simulink model "inAndOut_25b"  (R2025b)
settings: Solver=VariableStepAuto  AbsTol=1e-3
undefined symbols (not defined in the file or in its folder): ee_sli_rtmsupport, gcbh
libraries: nesl_utility x8
settings Model: Creator=yifany  LastModifiedBy=yifany
settings SolverCC: AutoScaleAbsTol=off  AlgebraicLoopSolver=TrustRegion  MaxZcPerStep=1.0
settings DebuggingCC: UnconnectedInputMsg=warning  UnconnectedOutputMsg=warning  UnconnectedLineMsg=warning  SymbolicDimsDataTypeCodeGenerationDiagnostic=none
settings ModelReferenceCC: EnableRefExpFcnMdlSchedulingChecks=on
settings SFSimCC: CustomCodeUndefinedFunction=UseInterfaceOnly
settings RTWCC: GPUComputeCapability=3.5  DLArmComputeVersion=19.05
settings SimscapeCC: SimscapeLogType=all  SimscapeLogSimulationStatistics=on  SimscapeLogDataHistory=10000.0

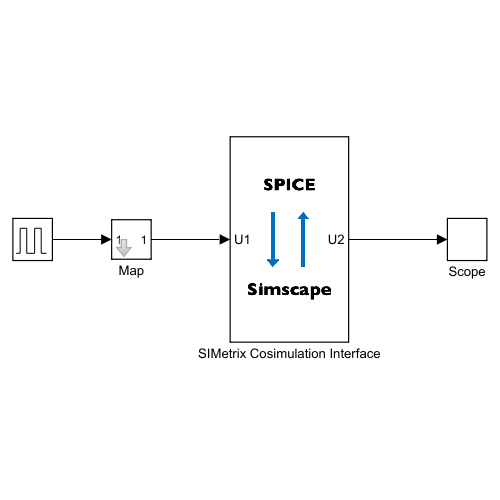
[thumbnail: Simulink's stored preview of the top-level diagram]
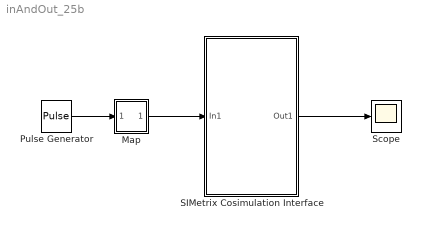
== system inAndOut_25b ==
  Map : Subsystem  mask{mapInput0=-8, mapInput1=25}
      mask prompts: mapInput0 "Map input 0 to output"; mapInput1 "Map input 1 to output"
      mask DialogControl DescTextVar Prompt: Linear map the input to the output
      mask DialogControl map Prompt: Map
  Pulse Generator : DiscretePulseGenerator  PulseType=Time based  Period=0.1  PulseWidth=40
  SIMetrix Cosimulation Interface : Subsystem  LoadFcn=ee_sli_rtmsupport( 'loadfcn', gcbh );  InitFcn=|  mask(SIMetrix Co-Simulation Interface){netlistFilePath=C:\Users\yifany\OneDrive - MathWorks\Desktop\Co-simulation\25b\inAndOut.net, flagGenerateInterface=1, numInputs=6, numOutputs=0, numVoltage=3, numCurrent=0, sampleTime=1e-3, updateIcon=1, DLLPath=C:\Program Files\SIMetrix910\bin64\Slif.dll}
      | % Checks Windows and sets the DLL path
      | ee.spice.internal.setDLLPathForWindows(gcb)
      mask prompts: netlistFilePath "physmod:ee:cosimulation:NetlistFilePath_MP"; numInputs "Number of simulink input signals"; numOutputs "Number of simulink output signals"; numVoltage "Number of voltage source electrical ports"; numCurrent "Number of current source electrical ports"; sampleTime "physmod:ee:cosimulation:SampleTime_MP"; updateIcon "Update Icon"; DLLPath "DLL path"
      mask help: physmod:ee:cosimulation:SimetrixCosimulationInterfacesBlock_MD
      mask init:
      | % Create the mask obj
      | maskObj = ee.spice.mask.cosimSIMetrix(gcb);
      | % Build IO
      | maskObj.buildIO;
      settings: DeleteFcn=ee_sli_rtmsupport( 'deletefcn', gcbh );  ModelCloseFcn=ee_sli_rtmsupport( 'modelclosefcn', gcbh );  PostSaveFcn=ee_sli_rtmsupport( 'postsavefcn', gcbh );  PreCopyFcn=ee_sli_rtmsupport( 'precopyfcn', gcbh );  OpenFcn=ee_sli_rtmsupport( 'openfcn', gcbh );  CloseFcn=ee_sli_rtmsupport( 'closefcn', gcbh );  PreDeleteFcn=ee_sli_rtmsupport( 'predeletefcn', gcbh );
      settings: CopyFcn=|
      | set_param(gcb,'LinkStatus','none')
      | ee_sli_rtmsupport( 'copyfcn', gcbh );
      mask Help: web([docroot '/sps/ref/simetrixcosimulationinterface.html'])
      mask DialogControl netlistFilePath Prompt: Netlist file path
      mask DialogControl BrowseBtn Prompt: physmod:ee:cosimulation:Browse_MP
      mask DialogControl BrowseBtn Callback:
      | % Create the mask obj
      | maskObj = ee.spice.mask.cosimSIMetrix(gcb);
      | % Browse netlist path
      | maskObj.browseNetlistPath;
      mask DialogControl buildIO Prompt: physmod:ee:cosimulation:BuildIO_MP
      mask DialogControl buildIO Callback:
      | blockObj = get_param(gcb,'Object');
      | dlg = DAStudio.ToolRoot.getOpenDialogs(blockObj.getDialogSource);
      | if ~isempty(dlg)
      |     dlg.apply;
      | end
      mask DialogControl numIO Prompt: I/O number
      mask DialogControl sampleTime Prompt: Sample time
      mask Display:
      | image('cosimSIMetrix.svg');
      | 
      | % Get parameters
      | updateIcon = str2double(get_param(gcb, 'updateIcon'));
      | netlistFilePath = get_param(gcb, 'netlistFilePath');
      | 
      | % Get interface port information from the netlist
      | if updateIcon
      |     netlistObj = ee.spice.internal.interfacePortInfo(netlistFilePath);
      |      % Get port information from the netlsit
      |      netlistObj = netlistObj.getPortsFromNetlist;
      | else
      |     netlistObj = ee.spice.internal.interfacePortInfo([]);
      | end
      | 
      | % Interface port handle
      | portHandles = get_param(gcb, 'PortHandles');
      | 
      | % Add input label
      | % Number of interface inport
      | numInport = length(portHandles.Inport);
      | for ii = 1:netlistObj.NumberOfInputs
      |     portName = upper(netlistObj.InputPortName(ii));
      |     if ii <= numInport
      |         port_label('input', ii, portName);
      |     end
      | end
      | 
      | % Add output label
      | % Number of interface outport
      | numOutport = length(portHandles.Outport);
      | for ii = 1:netlistObj.NumberOfOutputs
      |     portName = upper(netlistObj.OutputPortName(ii));
      |     if ii <= numOutport
      |         port_label('output', ii, portName);
      |     end
      | end
      | 
      | % Number of electrical connection port
      | numConnection = length(portHandles.RConn);
      | 
      | % Add voltage source electrical node
      | portIndex = 1;
      | for ii = 1:netlistObj.NumberOfVoltageSource
      |     portName = upper(netlistObj.VoltagePortName(ii));
      |     if netlistObj.VoltageIsDifferentialVector
      |         % Differential-end
      |         if portIndex + 1 <= numConnection
      |             port_label('rconn', portIndex, portName + "V +");
      |             port_label('rconn', portIndex + 1, portName + "V -");
      |             portIndex = portIndex + 2;
      |         end
      |     else
      |         % Single-end
      |         if portIndex <= numConnection
      |             port_label('rconn', portIndex, portName + "V");
      |             portIndex = portIndex + 1;
      |         end
      |     end
      | end
      | 
      | % Add current source electrical node
      | for ii = 1:netlistObj.NumberOfCurrentSource
      |     portName = upper(netlistObj.CurrentPortName(ii));
      |     if netlistObj.CurrentIsDifferentialVector
      |         % Differential-end
      |         if portIndex + 1 <= numConnection
      |             port_label('rconn', portIndex, portName + "I +");
      |             port_label('rconn', portIndex + 1, portName + "I -");
      |             portIndex = portIndex + 2;
      |         end
      |     else
      |         % Single-end
      |         if portIndex <= numConnection
      |             port_label('rconn', portIndex, portName + "I");
      |             portIndex = portIndex + 1;
      |         end
      |     end
      | end
  Scope : Scope
      settings: ActiveDisplayYMinimum=-61.816763160075034  ActiveDisplayYMaximum=562.41300067487691
  wires:
  SIMetrix Cosimulation Interface/1(Out1) -> Scope/1
  Pulse Generator/1 -> Map/1(In1)
  Map/1(Out1) -> SIMetrix Cosimulation Interface/1(In1)

== system inAndOut_25b/Map ==
  In1 : Inport
  Bias : Bias  Bias=mapInput0  SaturateOnIntegerOverflow=off
  Gain : Gain  Gain=mapInput1-mapInput0
  Out1 : Outport
  wires:
  Bias/1 -> Out1/1
  Gain/1 -> Bias/1
  In1/1 -> Gain/1

== system inAndOut_25b/SIMetrix Cosimulation Interface ==
  In1 : Inport
  Differential-Ended Network Coupler : Subsystem  Commented=on  Variant=on  mask{isNetworkCoupler=on, isVoltage=1, sampleTime=sampleTime, numNodes=1, i0=0, v0=0}
      mask prompts: isNetworkCoupler "Is network coupler"; isVoltage "Source type (1=voltage,0=current)"; sampleTime "Sample time (s)"; numNodes "Electrical node array size"; i0 "Initial current (A)"; v0 "Initial voltage (V)"
      settings: PortSchema="{\"entries\":[{\"content\":{\"sides\":[{\"content\":{\"connectorIds\":[\"In1\",\"Out1\"]},\"type\":\"ConnectorPlacement.EquallySpacedRectSide\",\"uuid\":\"c5b0d662-d741-4fab-bdd1-a9a465f659d9\"},{\"content\":{\"connectorIds\":[\"RConn1\",\"RConn2\"],\"side\":\"RIGHT\"},\"type\":\"ConnectorPlacement.EquallySpacedRectSide\",\"uuid\":\"848af5b9-7b7a-436a-bf47-17010bd721d3\"},{\"content\":{\"side\":\"TOP\"},\"type\":\"ConnectorPlacement.EquallySpacedRectSide\",\"uuid\":\"f4ff35f8-3dfd-4ab3-8ede-deadd7697822\"}]},\"type\":\"ConnectorPlacement.EquallySpacedConnector\",\"uuid\":\"b98b5658-49ee-4ac6-ad55-f0a4b59e49ca\"}],\"packageUris\":[\"http://schema.mathworks.com/mf0/Connector/R2020b\"],\"version\":\"1.0\"}"
      mask DialogControl DescGroupVar Prompt: Differential-Ended Network Coupler
      mask DialogControl DescTextVar Prompt: Connect Simscape differential electrical node pair(s) to SPICE via a controlled source.
      mask DialogControl Main Prompt: Main
      mask DialogControl InitialConditions Prompt: Initial Conditions
  S-function Interface to SIMetrix : S-Function  FunctionName=callSIMetrixInterface  Parameters=sampleTime, numInputs , elementsInput, numOutputs, elementsOutput, netlistPath, DLLPath  SFunctionDeploymentMode=off  EnableBusSupport=off  mask{sampleTime=sampleTime, numInputs=1, elementsInput=1, numOutputs=1, elementsOutput=1, netlistPath=C:\Users\yifany\OneDrive - MathWorks\Desktop\Co-simulation\25b\inAndOut.net, DLLPath=C:\Program Files\SIMetrix910\bin64\Slif.dll}
      mask prompts: sampleTime "Sample time (s)"; numInputs "Number of input ports"; elementsInput "Number of elements in each input"; numOutputs "Number of output ports"; elementsOutput "Number of elements in each output"; netlistPath "Netlist file path"; DLLPath "DLL path"
      mask init:
      | label = char(['Sample Time = ' num2str(sampleTime) 's']);
      mask Display: disp(label);
  Single-Ended Network Coupler : Subsystem  Commented=on  Variant=on  mask{isNetworkCoupler=on, isVoltage=1, sampleTime=sampleTime, numNodes=1, i0=0, v0=0}
      mask prompts: isNetworkCoupler "Is network coupler"; isVoltage "Source type (1=voltage,0=current)"; sampleTime "Sample time (s)"; numNodes "Electrical node array size"; i0 "Initial current (A)"; v0 "Initial voltage (V)"
      settings: PortSchema="{\"entries\":[{\"content\":{\"sides\":[{\"content\":{\"connectorIds\":[\"In1\",\"Out1\"]},\"type\":\"ConnectorPlacement.EquallySpacedRectSide\",\"uuid\":\"c5b0d662-d741-4fab-bdd1-a9a465f659d9\"},{\"content\":{\"connectorIds\":[\"RConn1\"],\"side\":\"RIGHT\"},\"type\":\"ConnectorPlacement.EquallySpacedRectSide\",\"uuid\":\"848af5b9-7b7a-436a-bf47-17010bd721d3\"},{\"content\":{\"side\":\"TOP\"},\"type\":\"ConnectorPlacement.EquallySpacedRectSide\",\"uuid\":\"f4ff35f8-3dfd-4ab3-8ede-deadd7697822\"}]},\"type\":\"ConnectorPlacement.EquallySpacedConnector\",\"uuid\":\"b98b5658-49ee-4ac6-ad55-f0a4b59e49ca\"}],\"packageUris\":[\"http://schema.mathworks.com/mf0/Connector/R2020b\"],\"version\":\"1.0\"}"
      mask DialogControl DescGroupVar Prompt: Network Single-End Coupler
      mask DialogControl DescTextVar Prompt: Connect Simscape single-ended electrical node(s) to SPICE via a controlled source.
      mask DialogControl Main Prompt: Main
      mask DialogControl InitialConditions Prompt: Initial Conditions
  Out1 : Outport
  wires:
  In1/1 -> S-function Interface to SIMetrix/1
  S-function Interface to SIMetrix/1 -> Out1/1

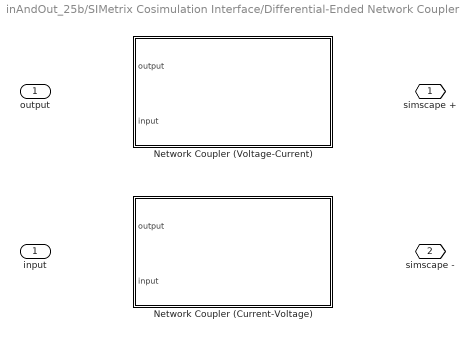
== system inAndOut_25b/SIMetrix Cosimulation Interface/Differential-Ended Network Coupler ==
  output : Inport
  Network Coupler (Current-Voltage) : Subsystem  VariantControl=isVoltage == 1  mask(SPICE-Simscape Interface (SPICE voltage source, Simscape current source)){h1=sampleTime, numNodes=numNodes, i0=i0, v0=v0}
      mask prompts: h1 "Sample time (s)"; numNodes "Electrical node array size"; i0 "Initial current (A)"; v0 "Initial voltage (V)"
      settings: PortSchema="{\"entries\":[{\"content\":{\"sides\":[{\"content\":{\"connectorIds\":[\"In1\",\"Out1\"]},\"type\":\"ConnectorPlacement.EquallySpacedRectSide\",\"uuid\":\"610a1ed6-b291-4a0b-a90d-70b8561de4e1\"},{\"content\":{\"connectorIds\":[\"RConn1\",\"RConn2\"],\"side\":\"RIGHT\"},\"type\":\"ConnectorPlacement.EquallySpacedRectSide\",\"uuid\":\"4485c82c-8fe2-4682-bcbc-6cb09abb17ba\"},{\"content\":{\"side\":\"TOP\"},\"type\":\"ConnectorPlacement.EquallySpacedRectSide\",\"uuid\":\"95b8fac6-4c79-4ea5-805e-3e8ec8ddf6c6\"}]},\"type\":\"ConnectorPlacement.EquallySpacedConnector\",\"uuid\":\"68c5dfd4-aae4-4799-81d8-d79fe9f653e9\"}],\"packageUris\":[\"http://schema.mathworks.com/mf0/Connector/R2020b\"],\"version\":\"1.0\"}"
      mask DialogControl Main Prompt: Main
      mask DialogControl InitialConditions Prompt: Initial Conditions
  Network Coupler (Voltage-Current) : Subsystem  VariantControl=isVoltage ~= 1  mask(SPICE-Simscape Interface (SPICE voltage source, Simscape current source)){h1=sampleTime, numNodes=numNodes, i0=i0, v0=v0}
      mask prompts: h1 "Sample time (s)"; numNodes "Electrical node array size"; i0 "Initial current (A)"; v0 "Initial voltage (V)"
      settings: PortSchema="{\"entries\":[{\"content\":{\"sides\":[{\"content\":{\"connectorIds\":[\"In1\",\"Out1\"]},\"type\":\"ConnectorPlacement.EquallySpacedRectSide\",\"uuid\":\"610a1ed6-b291-4a0b-a90d-70b8561de4e1\"},{\"content\":{\"connectorIds\":[\"RConn1\",\"RConn2\"],\"side\":\"RIGHT\"},\"type\":\"ConnectorPlacement.EquallySpacedRectSide\",\"uuid\":\"4485c82c-8fe2-4682-bcbc-6cb09abb17ba\"},{\"content\":{\"side\":\"TOP\"},\"type\":\"ConnectorPlacement.EquallySpacedRectSide\",\"uuid\":\"95b8fac6-4c79-4ea5-805e-3e8ec8ddf6c6\"}]},\"type\":\"ConnectorPlacement.EquallySpacedConnector\",\"uuid\":\"68c5dfd4-aae4-4799-81d8-d79fe9f653e9\"}],\"packageUris\":[\"http://schema.mathworks.com/mf0/Connector/R2020b\"],\"version\":\"1.0\"}"
      mask DialogControl Main Prompt: Main
      mask DialogControl InitialConditions Prompt: Initial Conditions
  simscape + : PMIOPort  Side=Right
  simscape - : PMIOPort  Port=2  Side=Right
  input : Outport

== system inAndOut_25b/SIMetrix Cosimulation Interface/Single-Ended Network Coupler ==
  output : Inport
  Network Coupler (Current-Voltage) : Subsystem  VariantControl=isVoltage == 1  mask(SPICE-Simscape Interface (SPICE voltage source, Simscape current source)){h1=sampleTime, numNodes=numNodes, i0=i0, v0=v0}
      mask prompts: h1 "Sample time (s)"; numNodes "Electrical node array size"; i0 "Initial current (A)"; v0 "Initial voltage (V)"
      settings: PortSchema="{\"entries\":[{\"content\":{\"sides\":[{\"content\":{\"connectorIds\":[\"In1\",\"Out1\"]},\"type\":\"ConnectorPlacement.EquallySpacedRectSide\",\"uuid\":\"610a1ed6-b291-4a0b-a90d-70b8561de4e1\"},{\"content\":{\"connectorIds\":[\"RConn1\"],\"side\":\"RIGHT\"},\"type\":\"ConnectorPlacement.EquallySpacedRectSide\",\"uuid\":\"4485c82c-8fe2-4682-bcbc-6cb09abb17ba\"},{\"content\":{\"side\":\"TOP\"},\"type\":\"ConnectorPlacement.EquallySpacedRectSide\",\"uuid\":\"95b8fac6-4c79-4ea5-805e-3e8ec8ddf6c6\"}]},\"type\":\"ConnectorPlacement.EquallySpacedConnector\",\"uuid\":\"68c5dfd4-aae4-4799-81d8-d79fe9f653e9\"}],\"packageUris\":[\"http://schema.mathworks.com/mf0/Connector/R2020b\"],\"version\":\"1.0\"}"
      mask DialogControl Main Prompt: Main
      mask DialogControl InitialConditions Prompt: Initial Conditions
  Network Coupler (Voltage-Current) : Subsystem  VariantControl=isVoltage ~= 1  mask(SPICE-Simscape Interface (SPICE voltage source, Simscape current source)){h1=sampleTime, numNodes=numNodes, i0=i0, v0=v0}
      mask prompts: h1 "Sample time (s)"; numNodes "Electrical node array size"; i0 "Initial current (A)"; v0 "Initial voltage (V)"
      settings: PortSchema="{\"entries\":[{\"content\":{\"sides\":[{\"content\":{\"connectorIds\":[\"In1\",\"Out1\"]},\"type\":\"ConnectorPlacement.EquallySpacedRectSide\",\"uuid\":\"610a1ed6-b291-4a0b-a90d-70b8561de4e1\"},{\"content\":{\"connectorIds\":[\"RConn1\"],\"side\":\"RIGHT\"},\"type\":\"ConnectorPlacement.EquallySpacedRectSide\",\"uuid\":\"4485c82c-8fe2-4682-bcbc-6cb09abb17ba\"},{\"content\":{\"side\":\"TOP\"},\"type\":\"ConnectorPlacement.EquallySpacedRectSide\",\"uuid\":\"95b8fac6-4c79-4ea5-805e-3e8ec8ddf6c6\"}]},\"type\":\"ConnectorPlacement.EquallySpacedConnector\",\"uuid\":\"68c5dfd4-aae4-4799-81d8-d79fe9f653e9\"}],\"packageUris\":[\"http://schema.mathworks.com/mf0/Connector/R2020b\"],\"version\":\"1.0\"}"
      mask DialogControl Main Prompt: Main
      mask DialogControl InitialConditions Prompt: Initial Conditions
  simscape : PMIOPort  Side=Right
  input : Outport

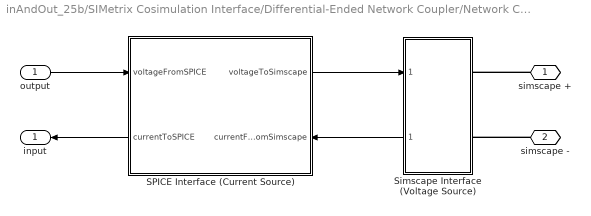
== system inAndOut_25b/SIMetrix Cosimulation Interface/Differential-Ended Network Coupler/Network Coupler (Current-Voltage) ==
  output : Inport
  SPICE Interface (Current Source) : Subsystem
      settings: PortSchema="{\"entries\":[{\"content\":{\"sides\":[{\"content\":{\"connectorIds\":[\"In1\",\"Out2\"]},\"type\":\"ConnectorPlacement.EquallySpacedRectSide\",\"uuid\":\"f9f70b4d-3b10-4b31-908f-8e396d51abf8\"},{\"content\":{\"connectorIds\":[\"Out1\",\"In2\"],\"side\":\"RIGHT\"},\"type\":\"ConnectorPlacement.EquallySpacedRectSide\",\"uuid\":\"ed689041-2a4d-4efe-8d21-4ea69e6c88bd\"},{\"content\":{\"side\":\"TOP\"},\"type\":\"ConnectorPlacement.EquallySpacedRectSide\",\"uuid\":\"15390e73-9972-43ef-8ad1-a6fecbf1c303\"}]},\"type\":\"ConnectorPlacement.EquallySpacedConnector\",\"uuid\":\"c13daa76-92fe-4d5b-a5f2-13005c05e77b\"}],\"packageUris\":[\"http://schema.mathworks.com/mf0/Connector/R2020b\"],\"version\":\"1.0\"}"
  Simscape Interface (Voltage Source) : Subsystem  mask{numNodes=numNodes}
      mask prompts: numNodes "Electrical node array size"
      settings: PortSchema="{\"entries\":[{\"content\":{\"sides\":[{\"content\":{\"connectorIds\":[\"In1\",\"Out1\"]},\"type\":\"ConnectorPlacement.EquallySpacedRectSide\",\"uuid\":\"5a4c1550-e77d-42df-bf3e-b81963920de7\"},{\"content\":{\"connectorIds\":[\"RConn1\",\"RConn2\"],\"side\":\"RIGHT\"},\"type\":\"ConnectorPlacement.EquallySpacedRectSide\",\"uuid\":\"3fd730f7-5937-4563-a365-595aaae9027b\"},{\"content\":{\"side\":\"TOP\"},\"type\":\"ConnectorPlacement.EquallySpacedRectSide\",\"uuid\":\"c16e04e4-26e8-4fd6-98d3-59adbef44c0d\"}]},\"type\":\"ConnectorPlacement.EquallySpacedConnector\",\"uuid\":\"5588d8d0-d459-45fe-a303-1ca6654e99d0\"}],\"packageUris\":[\"http://schema.mathworks.com/mf0/Connector/R2020b\"],\"version\":\"1.0\"}"
  simscape + : PMIOPort  Side=Right
  simscape - : PMIOPort  Port=2  Side=Right
  input : Outport
  wires:
  SPICE Interface (Current Source)/1(voltageToSimscape) -> Simscape Interface (Voltage Source)/1(voltage)
  output/1 -> SPICE Interface (Current Source)/1(voltageFromSPICE)
  SPICE Interface (Current Source)/2(currentToSPICE) -> input/1
  Simscape Interface (Voltage Source)/1(current) -> SPICE Interface (Current Source)/2(currentFromSimscape)
  connections:
  simscape +/RConn1 -- Simscape Interface (Voltage Source)/RConn1
  simscape -/RConn1 -- Simscape Interface (Voltage Source)/RConn2

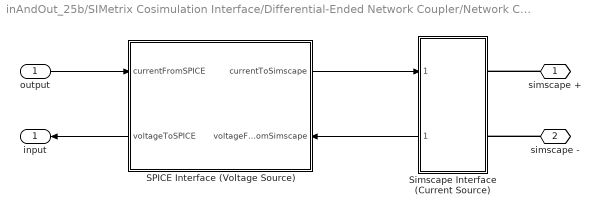
== system inAndOut_25b/SIMetrix Cosimulation Interface/Differential-Ended Network Coupler/Network Coupler (Voltage-Current) ==
  output : Inport
  SPICE Interface (Voltage Source) : Subsystem
      settings: PortSchema="{\"entries\":[{\"content\":{\"sides\":[{\"content\":{\"connectorIds\":[\"In1\",\"Out2\"]},\"type\":\"ConnectorPlacement.EquallySpacedRectSide\",\"uuid\":\"448ff72d-cc9d-4ea2-a4b3-f2ad8a335a2d\"},{\"content\":{\"connectorIds\":[\"Out1\",\"In2\"],\"side\":\"RIGHT\"},\"type\":\"ConnectorPlacement.EquallySpacedRectSide\",\"uuid\":\"1b2a7d42-0928-421d-bd53-992c9ec7cf4d\"},{\"content\":{\"side\":\"TOP\"},\"type\":\"ConnectorPlacement.EquallySpacedRectSide\",\"uuid\":\"0ddfa131-2eaa-4005-b3a1-aec50fa701a1\"}]},\"type\":\"ConnectorPlacement.EquallySpacedConnector\",\"uuid\":\"10303737-6ef5-489a-a2d1-9fada6e47834\"}],\"packageUris\":[\"http://schema.mathworks.com/mf0/Connector/R2020b\"],\"version\":\"1.0\"}"
  Simscape Interface (Current Source) : Subsystem  mask{numNodes=numNodes}
      mask prompts: numNodes "Electrical node array size"
      settings: PortSchema="{\"entries\":[{\"content\":{\"sides\":[{\"content\":{\"connectorIds\":[\"In1\",\"Out1\"]},\"type\":\"ConnectorPlacement.EquallySpacedRectSide\",\"uuid\":\"5a4c1550-e77d-42df-bf3e-b81963920de7\"},{\"content\":{\"connectorIds\":[\"RConn1\",\"RConn2\"],\"side\":\"RIGHT\"},\"type\":\"ConnectorPlacement.EquallySpacedRectSide\",\"uuid\":\"3fd730f7-5937-4563-a365-595aaae9027b\"},{\"content\":{\"side\":\"TOP\"},\"type\":\"ConnectorPlacement.EquallySpacedRectSide\",\"uuid\":\"c16e04e4-26e8-4fd6-98d3-59adbef44c0d\"}]},\"type\":\"ConnectorPlacement.EquallySpacedConnector\",\"uuid\":\"5588d8d0-d459-45fe-a303-1ca6654e99d0\"}],\"packageUris\":[\"http://schema.mathworks.com/mf0/Connector/R2020b\"],\"version\":\"1.0\"}"
  simscape + : PMIOPort  Side=Right
  simscape - : PMIOPort  Port=2  Side=Right
  input : Outport
  wires:
  Simscape Interface (Current Source)/1(voltage) -> SPICE Interface (Voltage Source)/2(voltageFromSimscape)
  SPICE Interface (Voltage Source)/2(voltageToSPICE) -> input/1
  output/1 -> SPICE Interface (Voltage Source)/1(currentFromSPICE)
  SPICE Interface (Voltage Source)/1(currentToSimscape) -> Simscape Interface (Current Source)/1(current)
  connections:
  simscape +/RConn1 -- Simscape Interface (Current Source)/RConn1
  simscape -/RConn1 -- Simscape Interface (Current Source)/RConn2

== system inAndOut_25b/SIMetrix Cosimulation Interface/Single-Ended Network Coupler/Network Coupler (Current-Voltage) ==
  output : Inport
  SPICE Interface (Current Source) : Subsystem
      settings: PortSchema="{\"entries\":[{\"content\":{\"sides\":[{\"content\":{\"connectorIds\":[\"In1\",\"Out2\"]},\"type\":\"ConnectorPlacement.EquallySpacedRectSide\",\"uuid\":\"f9f70b4d-3b10-4b31-908f-8e396d51abf8\"},{\"content\":{\"connectorIds\":[\"Out1\",\"In2\"],\"side\":\"RIGHT\"},\"type\":\"ConnectorPlacement.EquallySpacedRectSide\",\"uuid\":\"ed689041-2a4d-4efe-8d21-4ea69e6c88bd\"},{\"content\":{\"side\":\"TOP\"},\"type\":\"ConnectorPlacement.EquallySpacedRectSide\",\"uuid\":\"15390e73-9972-43ef-8ad1-a6fecbf1c303\"}]},\"type\":\"ConnectorPlacement.EquallySpacedConnector\",\"uuid\":\"c13daa76-92fe-4d5b-a5f2-13005c05e77b\"}],\"packageUris\":[\"http://schema.mathworks.com/mf0/Connector/R2020b\"],\"version\":\"1.0\"}"
  Simscape Interface (Voltage Source) : Subsystem  mask{numNodes=numNodes}
      mask prompts: numNodes "Electrical node array size"
      settings: PortSchema="{\"entries\":[{\"content\":{\"sides\":[{\"content\":{\"connectorIds\":[\"In1\",\"Out1\"]},\"type\":\"ConnectorPlacement.EquallySpacedRectSide\",\"uuid\":\"5a4c1550-e77d-42df-bf3e-b81963920de7\"},{\"content\":{\"connectorIds\":[\"RConn1\"],\"side\":\"RIGHT\"},\"type\":\"ConnectorPlacement.EquallySpacedRectSide\",\"uuid\":\"3fd730f7-5937-4563-a365-595aaae9027b\"},{\"content\":{\"connectorIds\":[],\"side\":\"TOP\"},\"type\":\"ConnectorPlacement.EquallySpacedRectSide\",\"uuid\":\"c16e04e4-26e8-4fd6-98d3-59adbef44c0d\"}]},\"type\":\"ConnectorPlacement.EquallySpacedConnector\",\"uuid\":\"5588d8d0-d459-45fe-a303-1ca6654e99d0\"}],\"packageUris\":[\"http://schema.mathworks.com/mf0/Connector/R2020b\"],\"version\":\"1.0\"}"
  simscape : PMIOPort  Side=Right
  input : Outport
  wires:
  SPICE Interface (Current Source)/2(currentToSPICE) -> input/1
  output/1 -> SPICE Interface (Current Source)/1(voltageFromSPICE)
  Simscape Interface (Voltage Source)/1(current) -> SPICE Interface (Current Source)/2(currentFromSimscape)
  SPICE Interface (Current Source)/1(voltageToSimscape) -> Simscape Interface (Voltage Source)/1(voltage)
  connections:
  simscape/RConn1 -- Simscape Interface (Voltage Source)/RConn1

== system inAndOut_25b/SIMetrix Cosimulation Interface/Single-Ended Network Coupler/Network Coupler (Voltage-Current) ==
  output : Inport
  SPICE Interface (Voltage Source) : Subsystem
      settings: PortSchema="{\"entries\":[{\"content\":{\"sides\":[{\"content\":{\"connectorIds\":[\"In1\",\"Out2\"]},\"type\":\"ConnectorPlacement.EquallySpacedRectSide\",\"uuid\":\"448ff72d-cc9d-4ea2-a4b3-f2ad8a335a2d\"},{\"content\":{\"connectorIds\":[\"Out1\",\"In2\"],\"side\":\"RIGHT\"},\"type\":\"ConnectorPlacement.EquallySpacedRectSide\",\"uuid\":\"1b2a7d42-0928-421d-bd53-992c9ec7cf4d\"},{\"content\":{\"side\":\"TOP\"},\"type\":\"ConnectorPlacement.EquallySpacedRectSide\",\"uuid\":\"0ddfa131-2eaa-4005-b3a1-aec50fa701a1\"}]},\"type\":\"ConnectorPlacement.EquallySpacedConnector\",\"uuid\":\"10303737-6ef5-489a-a2d1-9fada6e47834\"}],\"packageUris\":[\"http://schema.mathworks.com/mf0/Connector/R2020b\"],\"version\":\"1.0\"}"
  Simscape Interface (Current Source) : Subsystem  mask{numNodes=numNodes}
      mask prompts: numNodes "Electrical node array size"
      settings: PortSchema="{\"entries\":[{\"content\":{\"sides\":[{\"content\":{\"connectorIds\":[\"In1\",\"Out1\"]},\"type\":\"ConnectorPlacement.EquallySpacedRectSide\",\"uuid\":\"5a4c1550-e77d-42df-bf3e-b81963920de7\"},{\"content\":{\"connectorIds\":[\"RConn1\"],\"side\":\"RIGHT\"},\"type\":\"ConnectorPlacement.EquallySpacedRectSide\",\"uuid\":\"3fd730f7-5937-4563-a365-595aaae9027b\"},{\"content\":{\"connectorIds\":[],\"side\":\"TOP\"},\"type\":\"ConnectorPlacement.EquallySpacedRectSide\",\"uuid\":\"c16e04e4-26e8-4fd6-98d3-59adbef44c0d\"}]},\"type\":\"ConnectorPlacement.EquallySpacedConnector\",\"uuid\":\"5588d8d0-d459-45fe-a303-1ca6654e99d0\"}],\"packageUris\":[\"http://schema.mathworks.com/mf0/Connector/R2020b\"],\"version\":\"1.0\"}"
  simscape : PMIOPort  Side=Right
  input : Outport
  wires:
  SPICE Interface (Voltage Source)/1(currentToSimscape) -> Simscape Interface (Current Source)/1(current)
  output/1 -> SPICE Interface (Voltage Source)/1(currentFromSPICE)
  SPICE Interface (Voltage Source)/2(voltageToSPICE) -> input/1
  Simscape Interface (Current Source)/1(voltage) -> SPICE Interface (Voltage Source)/2(voltageFromSimscape)
  connections:
  simscape/RConn1 -- Simscape Interface (Current Source)/RConn1

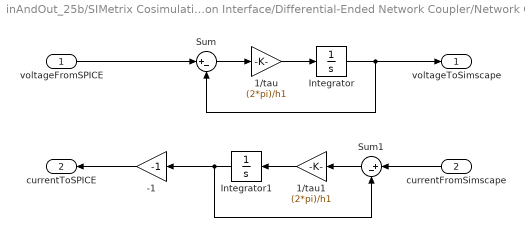
== system inAndOut_25b/SIMetrix Cosimulation Interface/Differential-Ended Network Coupler/Network Coupler (Current-Voltage)/SPICE Interface (Current Source) ==
  voltageFromSPICE : Inport
  currentFromSimscape : Inport  Port=2
  -1 : Gain  Gain=-1  SaturateOnIntegerOverflow=on  OutDataTypeStr=Inherit: Same as input  ParamDataTypeStr=Inherit: Same as input
  1/tau : Gain  Gain=(2*pi)/h1  SaturateOnIntegerOverflow=on  OutDataTypeStr=Inherit: Same as input  ParamDataTypeStr=Inherit: Same as input
  1/tau1 : Gain  Gain=(2*pi)/h1  SaturateOnIntegerOverflow=on  OutDataTypeStr=Inherit: Same as input  ParamDataTypeStr=Inherit: Same as input
  Integrator : Integrator  InitialCondition=v0
  Integrator1 : Integrator  InitialCondition=i0
  Sum : Sum  Inputs=|+-  InputSameDT=on  SaturateOnIntegerOverflow=on  OutDataTypeStr=Inherit: Same as first input
  Sum1 : Sum  Inputs=|+-  InputSameDT=on  SaturateOnIntegerOverflow=on  OutDataTypeStr=Inherit: Same as first input
  voltageToSimscape : Outport
  currentToSPICE : Outport  Port=2
  wires:
  -1/1 -> currentToSPICE/1
  Sum1/1 -> 1/tau1/1
  voltageFromSPICE/1 -> Sum/1
  1/tau/1 -> Integrator/1
  Integrator1/1 -> Sum1/2, -1/1
  Integrator/1 -> voltageToSimscape/1, Sum/2
  currentFromSimscape/1 -> Sum1/1
  Sum/1 -> 1/tau/1
  1/tau1/1 -> Integrator1/1

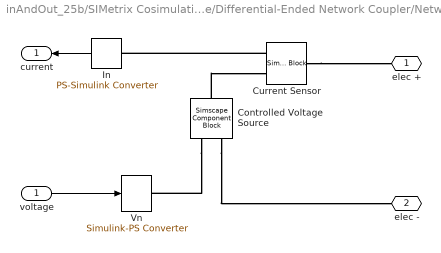
== system inAndOut_25b/SIMetrix Cosimulation Interface/Differential-Ended Network Coupler/Network Coupler (Current-Voltage)/Simscape Interface (Voltage Source) ==
  voltage : Inport
  Controlled Voltage Source : SimscapeComponentBlock  SourceFile=foundation.internal.couplers.electrical.voltageSource  ComponentPath=foundation.internal.couplers.electrical.voltageSource  ComponentVariants="[\"foundation.internal.couplers.electrical.voltageSource\"]"  ComponentVariantNames="[\"voltageSource\"]"  ClassName=voltageSource  SchemaVersion=1  threePhase=false  numNodes=numNodes
      settings: CopyFcn=simscape.sscblock.internal.componentBlockCallback(gcbh,'COPY')  PreCopyFcn=simscape.sscblock.internal.componentBlockCallback(gcbh,'PRECOPY')  PreDeleteFcn=simscape.sscblock.internal.componentBlockCallback(gcbh,'PREDELETE')
      mask Type: Controlled Voltage Source
  Current Sensor : SimscapeComponentBlock  SourceFile=foundation.internal.couplers.electrical.currentSensor  ComponentPath=foundation.internal.couplers.electrical.currentSensor  ComponentVariants="[\"foundation.internal.couplers.electrical.currentSensor\"]"  ComponentVariantNames="[\"currentSensor\"]"  ClassName=currentSensor  SchemaVersion=1  threePhase=false  numNodes=numNodes
      settings: CopyFcn=simscape.sscblock.internal.componentBlockCallback(gcbh,'COPY')  PreCopyFcn=simscape.sscblock.internal.componentBlockCallback(gcbh,'PRECOPY')  PreDeleteFcn=simscape.sscblock.internal.componentBlockCallback(gcbh,'PREDELETE')
      mask Type: Current Sensor
  In : nesl_utility/PS-Simulink Converter  PhysicalDomain=network_engine_domain  SubClassName=ps_output  LeftPortType=input  RightPortType=output  PseudoPeriodic=off  Frequencies=[]  VectorFormat=1-D array  Unit=A  AffineConversion=off
  Vn : nesl_utility/Simulink-PS Converter  PhysicalDomain=network_engine_domain  SubClassName=ps_input  LeftPortType=input  RightPortType=output  PseudoPeriodic=off  Frequencies=[]  NoiseDistribution=none  NoiseParameters=[]  Unit=V  AffineConversion=off  FilteringAndDerivatives=zero  SimscapeFilterOrder=1  InputFilterTimeConstant=0.001  UdotUserProvided=1
  elec + : PMIOPort  Side=Right
  elec - : PMIOPort  Port=2  Side=Right
  current : Outport
  wires:
  In/1 -> current/1
  voltage/1 -> Vn/1
  connections:
  Controlled Voltage Source/RConn1 -- Vn/RConn1
  Controlled Voltage Source/LConn1 -- Current Sensor/RConn2
  Current Sensor/LConn1 -- elec +/RConn1
  Current Sensor/RConn1 -- In/LConn1
  Controlled Voltage Source/RConn2 -- elec -/RConn1

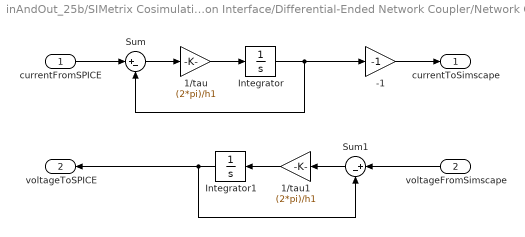
== system inAndOut_25b/SIMetrix Cosimulation Interface/Differential-Ended Network Coupler/Network Coupler (Voltage-Current)/SPICE Interface (Voltage Source) ==
  currentFromSPICE : Inport
  voltageFromSimscape : Inport  Port=2
  -1 : Gain  Gain=-1  SaturateOnIntegerOverflow=on  OutDataTypeStr=Inherit: Same as input  ParamDataTypeStr=Inherit: Same as input
  1/tau : Gain  Gain=(2*pi)/h1  SaturateOnIntegerOverflow=on  OutDataTypeStr=Inherit: Same as input  ParamDataTypeStr=Inherit: Same as input
  1/tau1 : Gain  Gain=(2*pi)/h1  SaturateOnIntegerOverflow=on  OutDataTypeStr=Inherit: Same as input  ParamDataTypeStr=Inherit: Same as input
  Integrator : Integrator  InitialCondition=v0
  Integrator1 : Integrator  InitialCondition=i0
  Sum : Sum  Inputs=|+-  InputSameDT=on  SaturateOnIntegerOverflow=on  OutDataTypeStr=Inherit: Same as first input
  Sum1 : Sum  Inputs=|+-  InputSameDT=on  SaturateOnIntegerOverflow=on  OutDataTypeStr=Inherit: Same as first input
  currentToSimscape : Outport
  voltageToSPICE : Outport  Port=2
  wires:
  -1/1 -> currentToSimscape/1
  currentFromSPICE/1 -> Sum/1
  1/tau1/1 -> Integrator1/1
  Sum/1 -> 1/tau/1
  voltageFromSimscape/1 -> Sum1/1
  Integrator/1 -> Sum/2, -1/1
  1/tau/1 -> Integrator/1
  Sum1/1 -> 1/tau1/1
  Integrator1/1 -> Sum1/2, voltageToSPICE/1

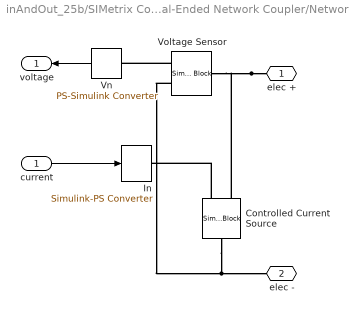
== system inAndOut_25b/SIMetrix Cosimulation Interface/Differential-Ended Network Coupler/Network Coupler (Voltage-Current)/Simscape Interface (Current Source) ==
  current : Inport
  Controlled Current Source : SimscapeComponentBlock  SourceFile=foundation.internal.couplers.electrical.currentSource  ComponentPath=foundation.internal.couplers.electrical.currentSource  ComponentVariants="[\"foundation.internal.couplers.electrical.currentSource\"]"  ComponentVariantNames="[\"currentSource\"]"  ClassName=currentSource  SchemaVersion=1  threePhase=false  numNodes=numNodes
      settings: CopyFcn=simscape.sscblock.internal.componentBlockCallback(gcbh,'COPY')  PreCopyFcn=simscape.sscblock.internal.componentBlockCallback(gcbh,'PRECOPY')  PreDeleteFcn=simscape.sscblock.internal.componentBlockCallback(gcbh,'PREDELETE')
      mask Type: Controlled Current Source
  In : nesl_utility/Simulink-PS Converter  PhysicalDomain=network_engine_domain  SubClassName=ps_input  LeftPortType=input  RightPortType=output  PseudoPeriodic=off  Frequencies=[]  NoiseDistribution=none  NoiseParameters=[]  Unit=A  AffineConversion=off  FilteringAndDerivatives=zero  SimscapeFilterOrder=1  InputFilterTimeConstant=0.001  UdotUserProvided=1
  Vn : nesl_utility/PS-Simulink Converter  PhysicalDomain=network_engine_domain  SubClassName=ps_output  LeftPortType=input  RightPortType=output  PseudoPeriodic=off  Frequencies=[]  VectorFormat=1-D array  Unit=V  AffineConversion=off
  Voltage Sensor : SimscapeComponentBlock  SourceFile=foundation.internal.couplers.electrical.voltageSensor  ComponentPath=foundation.internal.couplers.electrical.voltageSensor  ComponentVariants="[\"foundation.internal.couplers.electrical.voltageSensor\"]"  ComponentVariantNames="[\"voltageSensor\"]"  ClassName=voltageSensor  SchemaVersion=1  threePhase=false  numNodes=numNodes
      settings: CopyFcn=simscape.sscblock.internal.componentBlockCallback(gcbh,'COPY')  PreCopyFcn=simscape.sscblock.internal.componentBlockCallback(gcbh,'PRECOPY')  PreDeleteFcn=simscape.sscblock.internal.componentBlockCallback(gcbh,'PREDELETE')
      mask Type: Voltage Sensor
  elec + : PMIOPort  Side=Right
  elec - : PMIOPort  Port=2  Side=Right
  voltage : Outport
  wires:
  current/1 -> In/1
  Vn/1 -> voltage/1
  connections:
  Controlled Current Source/RConn1 -- In/RConn1
  Controlled Current Source/LConn1 -- Voltage Sensor/RConn2 -- elec -/RConn1
  Voltage Sensor/RConn1 -- Vn/LConn1
  elec +/RConn1 -- Controlled Current Source/RConn2 -- Voltage Sensor/LConn1

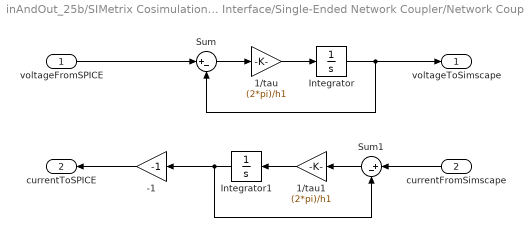
== system inAndOut_25b/SIMetrix Cosimulation Interface/Single-Ended Network Coupler/Network Coupler (Current-Voltage)/SPICE Interface (Current Source) ==
  voltageFromSPICE : Inport
  currentFromSimscape : Inport  Port=2
  -1 : Gain  Gain=-1  SaturateOnIntegerOverflow=on  OutDataTypeStr=Inherit: Same as input  ParamDataTypeStr=Inherit: Same as input
  1/tau : Gain  Gain=(2*pi)/h1  SaturateOnIntegerOverflow=on  OutDataTypeStr=Inherit: Same as input  ParamDataTypeStr=Inherit: Same as input
  1/tau1 : Gain  Gain=(2*pi)/h1  SaturateOnIntegerOverflow=on  OutDataTypeStr=Inherit: Same as input  ParamDataTypeStr=Inherit: Same as input
  Integrator : Integrator  InitialCondition=v0
  Integrator1 : Integrator  InitialCondition=i0
  Sum : Sum  Inputs=|+-  InputSameDT=on  SaturateOnIntegerOverflow=on  OutDataTypeStr=Inherit: Same as first input
  Sum1 : Sum  Inputs=|+-  InputSameDT=on  SaturateOnIntegerOverflow=on  OutDataTypeStr=Inherit: Same as first input
  voltageToSimscape : Outport
  currentToSPICE : Outport  Port=2
  wires:
  1/tau1/1 -> Integrator1/1
  Sum/1 -> 1/tau/1
  currentFromSimscape/1 -> Sum1/1
  Integrator/1 -> Sum/2, voltageToSimscape/1
  Integrator1/1 -> -1/1, Sum1/2
  1/tau/1 -> Integrator/1
  voltageFromSPICE/1 -> Sum/1
  Sum1/1 -> 1/tau1/1
  -1/1 -> currentToSPICE/1

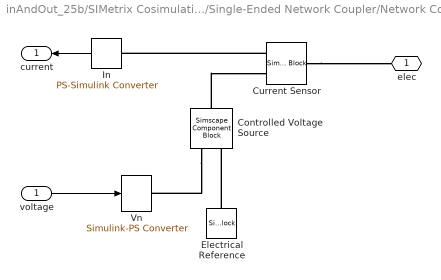
== system inAndOut_25b/SIMetrix Cosimulation Interface/Single-Ended Network Coupler/Network Coupler (Current-Voltage)/Simscape Interface (Voltage Source) ==
  voltage : Inport
  Controlled Voltage Source : SimscapeComponentBlock  SourceFile=foundation.internal.couplers.electrical.voltageSource  ComponentPath=foundation.internal.couplers.electrical.voltageSource  ComponentVariants="[\"foundation.internal.couplers.electrical.voltageSource\"]"  ComponentVariantNames="[\"voltageSource\"]"  ClassName=voltageSource  SchemaVersion=1  threePhase=false  numNodes=numNodes
      settings: CopyFcn=simscape.sscblock.internal.componentBlockCallback(gcbh,'COPY')  PreCopyFcn=simscape.sscblock.internal.componentBlockCallback(gcbh,'PRECOPY')  PreDeleteFcn=simscape.sscblock.internal.componentBlockCallback(gcbh,'PREDELETE')
      mask Type: Controlled Voltage Source
  Current Sensor : SimscapeComponentBlock  SourceFile=foundation.internal.couplers.electrical.currentSensor  ComponentPath=foundation.internal.couplers.electrical.currentSensor  ComponentVariants="[\"foundation.internal.couplers.electrical.currentSensor\"]"  ComponentVariantNames="[\"currentSensor\"]"  ClassName=currentSensor  SchemaVersion=1  threePhase=false  numNodes=numNodes
      settings: CopyFcn=simscape.sscblock.internal.componentBlockCallback(gcbh,'COPY')  PreCopyFcn=simscape.sscblock.internal.componentBlockCallback(gcbh,'PRECOPY')  PreDeleteFcn=simscape.sscblock.internal.componentBlockCallback(gcbh,'PREDELETE')
      mask Type: Current Sensor
  Electrical Reference : SimscapeComponentBlock  SourceFile=foundation.internal.couplers.electrical.reference  ComponentPath=foundation.internal.couplers.electrical.reference  ComponentVariants="[\"foundation.internal.couplers.electrical.reference\"]"  ComponentVariantNames="[\"reference\"]"  ClassName=reference  SchemaVersion=1  threePhase=false  numNodes=numNodes
      settings: CopyFcn=simscape.sscblock.internal.componentBlockCallback(gcbh,'COPY')  PreCopyFcn=simscape.sscblock.internal.componentBlockCallback(gcbh,'PRECOPY')  PreDeleteFcn=simscape.sscblock.internal.componentBlockCallback(gcbh,'PREDELETE')
      mask Type: Electrical Reference
  In : nesl_utility/PS-Simulink Converter  PhysicalDomain=network_engine_domain  SubClassName=ps_output  LeftPortType=input  RightPortType=output  PseudoPeriodic=off  Frequencies=[]  VectorFormat=1-D array  Unit=A  AffineConversion=off
  Vn : nesl_utility/Simulink-PS Converter  PhysicalDomain=network_engine_domain  SubClassName=ps_input  LeftPortType=input  RightPortType=output  PseudoPeriodic=off  Frequencies=[]  NoiseDistribution=none  NoiseParameters=[]  Unit=V  AffineConversion=off  FilteringAndDerivatives=zero  SimscapeFilterOrder=1  InputFilterTimeConstant=0.001  UdotUserProvided=1
  elec : PMIOPort  Side=Right
  current : Outport
  wires:
  voltage/1 -> Vn/1
  In/1 -> current/1
  connections:
  Electrical Reference/LConn1 -- Controlled Voltage Source/RConn2
  Current Sensor/RConn1 -- In/LConn1
  Current Sensor/LConn1 -- elec/RConn1
  Controlled Voltage Source/LConn1 -- Current Sensor/RConn2
  Controlled Voltage Source/RConn1 -- Vn/RConn1

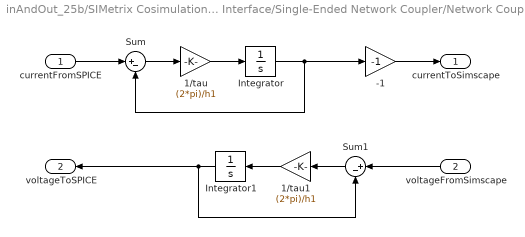
== system inAndOut_25b/SIMetrix Cosimulation Interface/Single-Ended Network Coupler/Network Coupler (Voltage-Current)/SPICE Interface (Voltage Source) ==
  currentFromSPICE : Inport
  voltageFromSimscape : Inport  Port=2
  -1 : Gain  Gain=-1  SaturateOnIntegerOverflow=on  OutDataTypeStr=Inherit: Same as input  ParamDataTypeStr=Inherit: Same as input
  1/tau : Gain  Gain=(2*pi)/h1  SaturateOnIntegerOverflow=on  OutDataTypeStr=Inherit: Same as input  ParamDataTypeStr=Inherit: Same as input
  1/tau1 : Gain  Gain=(2*pi)/h1  SaturateOnIntegerOverflow=on  OutDataTypeStr=Inherit: Same as input  ParamDataTypeStr=Inherit: Same as input
  Integrator : Integrator  InitialCondition=v0
  Integrator1 : Integrator  InitialCondition=i0
  Sum : Sum  Inputs=|+-  InputSameDT=on  SaturateOnIntegerOverflow=on  OutDataTypeStr=Inherit: Same as first input
  Sum1 : Sum  Inputs=|+-  InputSameDT=on  SaturateOnIntegerOverflow=on  OutDataTypeStr=Inherit: Same as first input
  currentToSimscape : Outport
  voltageToSPICE : Outport  Port=2
  wires:
  Integrator1/1 -> voltageToSPICE/1, Sum1/2
  Sum1/1 -> 1/tau1/1
  1/tau/1 -> Integrator/1
  Integrator/1 -> -1/1, Sum/2
  voltageFromSimscape/1 -> Sum1/1
  Sum/1 -> 1/tau/1
  1/tau1/1 -> Integrator1/1
  currentFromSPICE/1 -> Sum/1
  -1/1 -> currentToSimscape/1

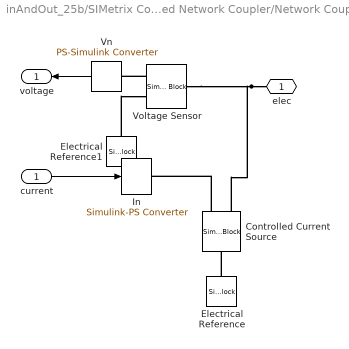
== system inAndOut_25b/SIMetrix Cosimulation Interface/Single-Ended Network Coupler/Network Coupler (Voltage-Current)/Simscape Interface (Current Source) ==
  current : Inport
  Controlled Current Source : SimscapeComponentBlock  SourceFile=foundation.internal.couplers.electrical.currentSource  ComponentPath=foundation.internal.couplers.electrical.currentSource  ComponentVariants="[\"foundation.internal.couplers.electrical.currentSource\"]"  ComponentVariantNames="[\"currentSource\"]"  ClassName=currentSource  SchemaVersion=1  threePhase=false  numNodes=numNodes
      settings: CopyFcn=simscape.sscblock.internal.componentBlockCallback(gcbh,'COPY')  PreCopyFcn=simscape.sscblock.internal.componentBlockCallback(gcbh,'PRECOPY')  PreDeleteFcn=simscape.sscblock.internal.componentBlockCallback(gcbh,'PREDELETE')
      mask Type: Controlled Current Source
  Electrical Reference : SimscapeComponentBlock  SourceFile=foundation.internal.couplers.electrical.reference  ComponentPath=foundation.internal.couplers.electrical.reference  ComponentVariants="[\"foundation.internal.couplers.electrical.reference\"]"  ComponentVariantNames="[\"reference\"]"  ClassName=reference  SchemaVersion=1  threePhase=false  numNodes=numNodes
      settings: CopyFcn=simscape.sscblock.internal.componentBlockCallback(gcbh,'COPY')  PreCopyFcn=simscape.sscblock.internal.componentBlockCallback(gcbh,'PRECOPY')  PreDeleteFcn=simscape.sscblock.internal.componentBlockCallback(gcbh,'PREDELETE')
      mask Type: Electrical Reference
  Electrical Reference1 : SimscapeComponentBlock  SourceFile=foundation.internal.couplers.electrical.reference  ComponentPath=foundation.internal.couplers.electrical.reference  ComponentVariants="[\"foundation.internal.couplers.electrical.reference\"]"  ComponentVariantNames="[\"reference\"]"  ClassName=reference  SchemaVersion=1  threePhase=false  numNodes=numNodes
      settings: CopyFcn=simscape.sscblock.internal.componentBlockCallback(gcbh,'COPY')  PreCopyFcn=simscape.sscblock.internal.componentBlockCallback(gcbh,'PRECOPY')  PreDeleteFcn=simscape.sscblock.internal.componentBlockCallback(gcbh,'PREDELETE')
      mask Type: Electrical Reference
  In : nesl_utility/Simulink-PS Converter  PhysicalDomain=network_engine_domain  SubClassName=ps_input  LeftPortType=input  RightPortType=output  PseudoPeriodic=off  Frequencies=[]  NoiseDistribution=none  NoiseParameters=[]  Unit=A  AffineConversion=off  FilteringAndDerivatives=zero  SimscapeFilterOrder=1  InputFilterTimeConstant=0.001  UdotUserProvided=1
  Vn : nesl_utility/PS-Simulink Converter  PhysicalDomain=network_engine_domain  SubClassName=ps_output  LeftPortType=input  RightPortType=output  PseudoPeriodic=off  Frequencies=[]  VectorFormat=1-D array  Unit=V  AffineConversion=off
  Voltage Sensor : SimscapeComponentBlock  SourceFile=foundation.internal.couplers.electrical.voltageSensor  ComponentPath=foundation.internal.couplers.electrical.voltageSensor  ComponentVariants="[\"foundation.internal.couplers.electrical.voltageSensor\"]"  ComponentVariantNames="[\"voltageSensor\"]"  ClassName=voltageSensor  SchemaVersion=1  threePhase=false  numNodes=numNodes
      settings: CopyFcn=simscape.sscblock.internal.componentBlockCallback(gcbh,'COPY')  PreCopyFcn=simscape.sscblock.internal.componentBlockCallback(gcbh,'PRECOPY')  PreDeleteFcn=simscape.sscblock.internal.componentBlockCallback(gcbh,'PREDELETE')
      mask Type: Voltage Sensor
  elec : PMIOPort  Side=Right
  voltage : Outport
  wires:
  Vn/1 -> voltage/1
  current/1 -> In/1
  connections:
  Electrical Reference1/LConn1 -- Voltage Sensor/RConn2
  elec/RConn1 -- Voltage Sensor/LConn1 -- Controlled Current Source/RConn2
  Voltage Sensor/RConn1 -- Vn/LConn1
  Electrical Reference/LConn1 -- Controlled Current Source/LConn1
  Controlled Current Source/RConn1 -- In/RConn1
